simulink model "CalcReturn"  (R2018b)
settings: Solver=FixedStepDiscrete  StartTime=0.0  StopTime=1000  FixedStep=0.1  RelTol=1e-3  EnableMultiTasking=on
libraries: GroupLib x4
settings Model: Creator=higashit  LastModifiedBy=tliang
settings SolverCC: AlgebraicLoopSolver=LineSearch
settings DataIOCC: LimitDataPoints=on  SaveFormat=Array  SaveOutput=off  SaveTime=off
settings OptimizationCC: ExpressionDepthLimit=2147483647  EfficientFloat2IntCast=on  LifeSpan=inf
settings DebuggingCC: SolverPrmCheckMsg=warning  UniqueDataStoreMsg=error  StateNameClashWarn=warning  LibraryContextMissingDiagnostic=none  StrictBusMsg=ErrorOnBusTreatedAsVector  SFUnexpectedBacktrackingDiag=warning  SFNoUnconditionalDefaultTransitionDiag=warning  SFExecutionAtInitializationDiag=none
settings HardwareCC: ProdBitPerPointer=32  ProdBitPerSizeT=32  ProdBitPerPtrDiffT=32  ProdLargestAtomicFloat=None  ProdIntDivRoundTo=Undefined  ProdEndianess=Unspecified  ProdWordSize=32  ProdHWDeviceType=32-bit Generic
settings ModelReferenceCC: PropagateSignalLabelsOutOfModel=off
settings SFSimCC: SimUseLocalCustomCode=off
settings RTWCC: RTWUseLocalCustomCode=off
settings CodeAppCC: StateflowObjectComments=on
settings GRTTargetCC: TargetLangStandard=C89/C90 (ANSI)  GeneratePreprocessorConditionals=Disable all
settings ConfigComp: CovMetricSettings=dw  CovHtmlReporting=on  CovSaveCumulativeToWorkspaceVar=on  CovSaveSingleToWorkspaceVar=on  CovExternalEMLEnable=off

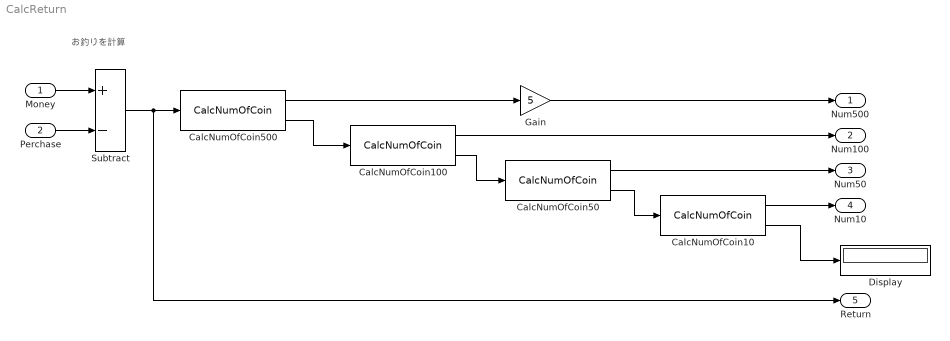
== system CalcReturn ==
  note: お釣りを計算
  Money : Inport  OutDataTypeStr=uint16  PortDimensions=1
  Perchase : Inport  Port=2  OutDataTypeStr=uint16  PortDimensions=1
  CalcNumOfCoin10 : GroupLib/CalcNumOfCoin  Coin=10
  CalcNumOfCoin100 : GroupLib/CalcNumOfCoin  Coin=100
  CalcNumOfCoin50 : GroupLib/CalcNumOfCoin  Coin=50
  CalcNumOfCoin500 : GroupLib/CalcNumOfCoin  Coin=500
  Display : Display
  Gain : Gain  Gain=5
  Subtract : Sum  Inputs=+-
  Num500 : Outport  OutDataTypeStr=uint16  PortDimensions=1
  Num100 : Outport  Port=2  OutDataTypeStr=uint16  PortDimensions=1
  Num50 : Outport  Port=3  OutDataTypeStr=uint16  PortDimensions=1
  Num10 : Outport  Port=4  OutDataTypeStr=uint16  PortDimensions=1
  Return : Outport  Port=5  OutDataTypeStr=uint16  PortDimensions=1
  wires:
  CalcNumOfCoin500/2 -> CalcNumOfCoin100/1
  CalcNumOfCoin100/2 -> CalcNumOfCoin50/1
  CalcNumOfCoin50/2 -> CalcNumOfCoin10/1
  Money/1 -> Subtract/1
  Perchase/1 -> Subtract/2
  Subtract/1 -> CalcNumOfCoin500/1, Return/1
  CalcNumOfCoin500/1 -> Gain/1
  CalcNumOfCoin100/1 -> Num100/1
  CalcNumOfCoin50/1 -> Num50/1
  CalcNumOfCoin10/1 -> Num10/1
  CalcNumOfCoin10/2 -> Display/1
  Gain/1 -> Num500/1
